simulink model "ClosedLoop"  (R2023b)
settings: Solver=ode1  StartTime=0.0  StopTime=inf  FixedStep=0.005  RelTol=1e-3  EnableMultiTasking=on
undefined symbols (not defined in the file or in its folder): Abar, Bbar, Cbar, F, G, Lbar
libraries: arduinolib x2, simulink x2
settings Model: SimulationMode=external  ExtModeTrigDuration=2  Creator=Alex  LastModifiedBy=jose
settings SolverCC: AlgebraicLoopSolver=TrustRegion
settings DataIOCC: SaveFormat=StructureWithTime  ReturnWorkspaceOutputs=off
settings OptimizationCC: PassReuseOutputArgsAs=Individual arguments  MaxStackSize=64  EfficientTunableParamExpr=on
settings DebuggingCC: ParameterTunabilityLossMsg=error  UnconnectedInputMsg=warning  UnconnectedOutputMsg=warning  UnconnectedLineMsg=warning  ArithmeticOperatorsInVariantConditions=warning
settings HardwareCC: ProdBitPerInt=16  ProdBitPerPointer=16  ProdBitPerSizeT=16  ProdBitPerPtrDiffT=16  ProdLargestAtomicFloat=None  ProdWordSize=8  ProdHWDeviceType=Atmel->AVR
settings ModelReferenceCC: EnableRefExpFcnMdlSchedulingChecks=on
settings SFSimCC: SimUseLocalCustomCode=off  MATLABDynamicMemAlloc=off  CustomCodeUndefinedFunction=UseInterfaceOnly
settings RTWCC: Description=Embedded Coder  SystemTargetFile=ert.tlc  HardwareBoard=Arduino Mega 2560  TemplateMakefile=ert_default_tmf  RTWUseLocalCustomCode=off  Toolchain=Arduino AVR  BuildConfiguration=Faster Runs  IncludeHyperlinkInReport=on  DLArmComputeVersion=19.05
settings CodeAppCC: ForceParamTrailComments=on  IgnoreCustomStorageClasses=off  OperatorAnnotations=on  SimulinkDataObjDesc=on  SFDataObjDesc=on  InsertBlockDesc=on
settings ERTTargetCC: SupportContinuousTime=on  SupportVariableSizeSignals=on  ExtModeTransport=3  ExtModeStaticAlloc=on  ExtModeStaticAllocSize=1000  ExtModeMexFile=ext_xcp  ExtModeIntrfLevel=Level2 - Open

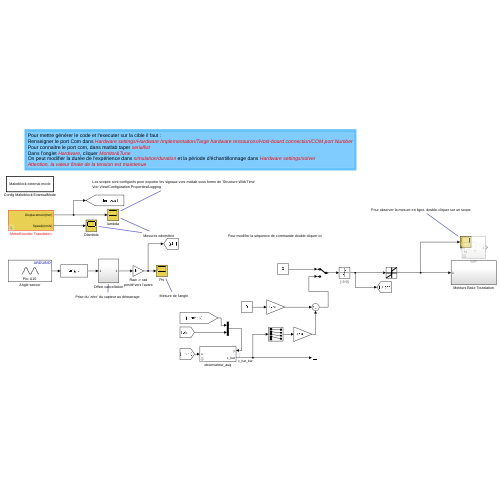
[thumbnail: Simulink's stored preview of the top-level diagram]
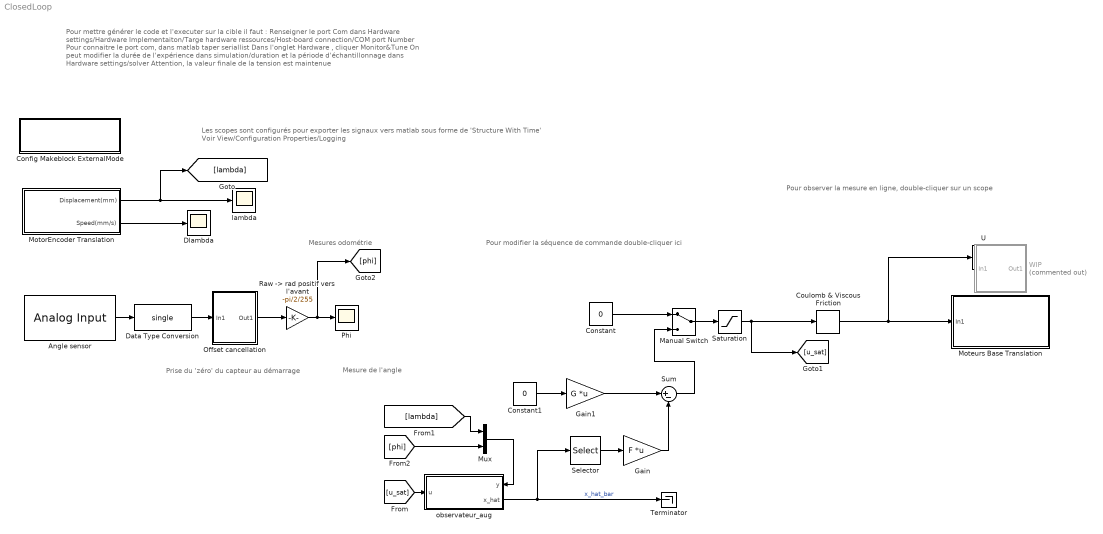
== system ClosedLoop ==
  note: Prise du 'zéro' du capteur au démarrage
  note: Mesure de l'angle
  note: Mesures odométrie
  note: Pour observer la mesure en ligne, double-cliquer sur un scope
  note: Pour modifier la séquence de commande double-cliquer ici
  note: Pour mettre générer le code et l'executer sur la cible il faut :
      | Renseigner le port Com dans Hardware settings/Hardware Implementaiton/Targe hardware ressources/Host-board connection/COM port Number
      | Pour connaitre le port com, dans matlab taper seriallist
      | Dans l'onglet Hardware , cliquer Monitor&Tune
      | On peut modifier la durée de l'expérience dans simulation/duration et la période d'échantillonnage dans Hardware settings/solver
      | Attention, la valeur finale de la tension est maintenue
  note: Les scopes sont configurés pour exporter les signaux vers matlab sous forme de 'Structure With Time'
      | Voir View/Configuration Properties/Logging
  Angle sensor : arduinolib/Analog Input  pinNumber=10  ReadResultsOnly=off  ConversionTriggerSource=Software  ExternalTriggerType=uint32(0)  OutputDataType=uint16  EnableConversionCompleteNotify=off  EnableOuputStatus=off  SampleTime=-1  blockPlatform=arduino
  Config Makeblock ExternalMode : Subsystem  LoadFcn=set_param(gcb,'MaskHideContents','on')  InitFcn=|  TreatAsAtomicUnit=on
      | codertarget.arduinobase.registry.setBaudRate(gcs,115200)
      | set_param(gcb,'MaskHideContents','on')
      mask Display: disp('Makeblock external mode')
  Constant : Constant  Value=0
  Constant1 : Constant  Value=0
  Coulomb & Viscous Friction : simulink/Discontinuities/Coulomb & Viscous Friction  offset=0.5  gain=1
  Data Type Conversion : DataTypeConversion  OutDataTypeStr=single  SaturateOnIntegerOverflow=off  RndMeth=Floor
  Dlambda : Scope
  Gain : Gain  Gain=F  Multiplication=Matrix(K*u)
  Gain1 : Gain  Gain=G  Multiplication=Matrix(K*u)
  Manual Switch : ManualSwitch
  Moteurs Base Translation : Subsystem
  MotorEncoder Translation : Subsystem  mask{pulsePerTurn=8, beltPitch=2.032, nTeeth=90, gearRatio=46}
      mask prompts: pulsePerTurn "Encoder resolution"; beltPitch "Belt Pitch"; nTeeth "Number of teeth"; gearRatio "Gear ratio"
  Mux : Mux  Inputs=2
  Offset cancellation : Subsystem
  Phi : Scope
  "Raw -> rad positif vers l'avant" : Gain  Gain=-pi/2/255
  Saturation : Saturate  UpperLimit=9  LowerLimit=-9
      settings: AttributesFormatString=[%<LowerLimit> %<UpperLimit>]
  Selector : Selector  InputPortWidth=5  IndexOptions=Index vector (dialog)  Indices=[1:4]  OutputSizes=1
  Sum : Sum  Inputs=|+-
  Terminator : Terminator
  U : Scope
  WIP : Subsystem  Commented=on
  lambda : Scope
  observateur_aug : Subsystem  mask{A=Abar, B=Bbar, C=Cbar, x_hat0=0, L=Lbar}
      mask prompts: A "Matrice A"; B "Matrice B"; C "Matrice C"; x_hat0 "Condition initiale"; L "gain L"
      settings: PortSchema="{\"entries\":[{\"content\":{\"sides\":[{\"content\":{\"connectorIds\":[\"In1\"]},\"type\":\"ConnectorPlacement.EquallySpacedRectSide\",\"uuid\":\"1c206b57-f343-4802-943f-f396b5f2fa44\"},{\"content\":{\"connectorIds\":[\"In2\",\"Out1\"],\"side\":\"RIGHT\"},\"type\":\"ConnectorPlacement.EquallySpacedRectSide\",\"uuid\":\"35da9abd-d6b1-4089-aae6-a46dbed03912\"},{\"content\":{\"connectorIds\":[],\"side\":\"TOP\"},\"type\":\"ConnectorPlacement.EquallySpacedRectSide\",\"uuid\":\"b9f72e83-9b94-44ec-a47d-5a0319960312\"}]},\"type\":\"ConnectorPlacement.EquallySpacedConnector\",\"uuid\":\"6461eadb-104c-4216-897a-8e335480794d\"}],\"packageUris\":[\"http://schema.mathworks.com/mf0/Connector/R2020b\"],\"version\":\"1.0\"}"
  wires:
  MotorEncoder Translation/1(Displacement(mm)) -> [lambda], lambda/1
  Saturation/1 -> [u_sat], Coulomb & Viscous Friction/1
  Constant/1 -> Manual Switch/1
  Angle sensor/1 -> Data Type Conversion/1
  Offset cancellation/1(Out1) -> "Raw -> rad positif vers l'avant"/1
  Data Type Conversion/1 -> Offset cancellation/1(In1)
  "Raw -> rad positif vers l'avant"/1 -> [phi], Phi/1
  MotorEncoder Translation/2(Speed(mm/s)) -> Dlambda/1
  Manual Switch/1 -> Saturation/1
  [u_sat] -> observateur_aug/1(u)
  [lambda] -> Mux/1
  [phi] -> Mux/2
  Mux/1 -> observateur_aug/2(y)
  observateur_aug/1(x_hat) -> Selector/1, Terminator/1  "x_hat_bar"
  Selector/1 -> Gain/1
  Gain1/1 -> Sum/1
  Constant1/1 -> Gain1/1
  Gain/1 -> Sum/2
  Sum/1 -> Manual Switch/2
  Coulomb & Viscous Friction/1 -> U/1, Moteurs Base Translation/1(In1)

== system ClosedLoop/Config Makeblock ExternalMode ==

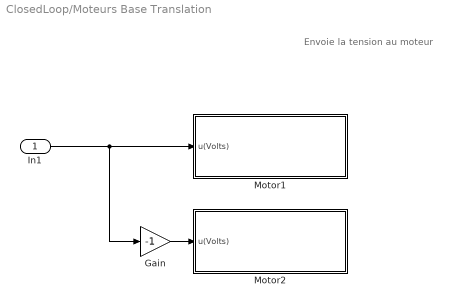
== system ClosedLoop/Moteurs Base Translation ==
  note: Envoie la tension au moteur
  In1 : Inport
  Gain : Gain  Gain=-1
  Motor1 : Subsystem  mask{Vmax=12}
      mask prompts: Vmax "Power supply Voltage"
  Motor2 : Subsystem  mask{Vmax=12}
      mask prompts: Vmax "Power supply Voltage"
  wires:
  Gain/1 -> Motor2/1(u(Volts))
  In1/1 -> Gain/1, Motor1/1(u(Volts))

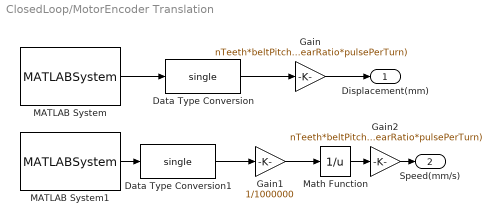
== system ClosedLoop/MotorEncoder Translation ==
  Data Type Conversion : DataTypeConversion  OutDataTypeStr=single  SaturateOnIntegerOverflow=off  RndMeth=Floor
  Data Type Conversion1 : DataTypeConversion  OutDataTypeStr=single  SaturateOnIntegerOverflow=off  RndMeth=Floor
  Gain : Gain  Gain=nTeeth*beltPitch/(gearRatio*pulsePerTurn)  OutDataTypeStr=single
      settings: AttributesFormatString=%<Gain>
  Gain1 : Gain  Gain=1/1000000
  Gain2 : Gain  Gain=nTeeth*beltPitch/(gearRatio*pulsePerTurn)  OutDataTypeStr=single
      settings: AttributesFormatString=%<Gain>
  MATLAB System : MATLABSystem  System=Enc1Read  SampleTime=-1
      mask Type: Enc1Read
      mask Display:
      | disp('Encoder 1');
      | port_label('output',1,'y');
  MATLAB System1 : MATLABSystem  System=Enc1Period  SampleTime=-1
      mask Type: Enc1Period
      mask Display:
      | disp('Encoder Period 1');
      | port_label('output',1,'y');
  Math Function : Math  Operator=reciprocal  SignedPower=on  OutputSignalType=real  OutDataTypeStr=single  SaturateOnIntegerOverflow=off
  Displacement(mm) : Outport  VectorParamsAs1DForOutWhenUnconnected=off
  Speed(mm/s) : Outport  Port=2  VectorParamsAs1DForOutWhenUnconnected=off
  wires:
  MATLAB System/1 -> Data Type Conversion/1
  Gain/1 -> Displacement(mm)/1
  Data Type Conversion/1 -> Gain/1
  Gain1/1 -> Math Function/1
  Data Type Conversion1/1 -> Gain1/1
  MATLAB System1/1 -> Data Type Conversion1/1
  Math Function/1 -> Gain2/1
  Gain2/1 -> Speed(mm/s)/1

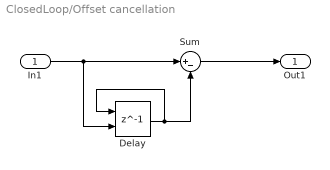
== system ClosedLoop/Offset cancellation ==
  In1 : Inport
  Delay : Delay  DelayLength=1  InitialConditionSource=Input port
      settings: InputPortMap=u0,p4
  Sum : Sum  Inputs=|+-
  Out1 : Outport  VectorParamsAs1DForOutWhenUnconnected=off
  wires:
  In1/1 -> Sum/1, Delay/2
  Delay/1 -> Sum/2, Delay/1
  Sum/1 -> Out1/1

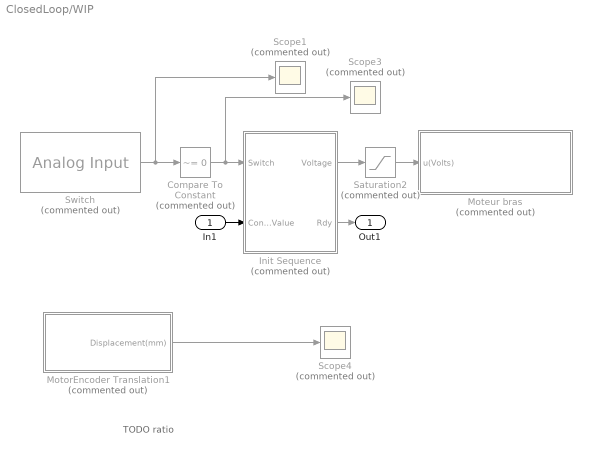
== system ClosedLoop/WIP ==
  note: TODO ratio
  In1 : Inport
  Compare To Constant : simulink/Logic and Bit Operations/Compare To Constant  Commented=on  relop=~=  const=0  OutDataTypeStr=boolean
  Init Sequence : Stateflow chart  Commented=on  TreatAsAtomicUnit=on
  Moteur bras : Subsystem  Commented=on  mask{Vmax=12}
      mask prompts: Vmax "Power supply Voltage"
  MotorEncoder Translation1 : Subsystem  Commented=on  mask{pulsePerTurn=8, beltPitch=2.032, nTeeth=90, gearRatio=46}
      mask prompts: pulsePerTurn "Encoder resolution"; beltPitch "Belt Pitch"; nTeeth "Number of teeth"; gearRatio "Gear ratio"
  Saturation2 : Saturate  Commented=on  UpperLimit=9  LowerLimit=-9
      settings: AttributesFormatString=[%<LowerLimit> %<UpperLimit>]
  Scope1 : Scope  Commented=on
  Scope3 : Scope  Commented=on
  Scope4 : Scope  Commented=on
  Switch : arduinolib/Analog Input  Commented=on  pinNumber=11  ReadResultsOnly=off  ConversionTriggerSource=Software  ExternalTriggerType=uint32(0)  OutputDataType=uint16  EnableConversionCompleteNotify=off  EnableOuputStatus=off  SampleTime=-1  blockPlatform=arduino
  Out1 : Outport
  wires:
  In1/1 -> Init Sequence/2(ControlValue)
  Init Sequence/1(Voltage) -> Saturation2/1
  Init Sequence/2(Rdy) -> Out1/1
  Switch/1 -> Scope1/1, Compare To Constant/1
  Compare To Constant/1 -> Scope3/1, Init Sequence/1(Switch)
  MotorEncoder Translation1/1(Displacement(mm)) -> Scope4/1
  Saturation2/1 -> Moteur bras/1(u(Volts))

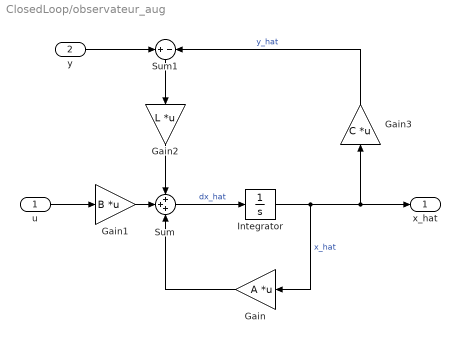
== system ClosedLoop/observateur_aug ==
  u : Inport
  y : Inport  Port=2
  Gain : Gain  Gain=A  Multiplication=Matrix(K*u)
  Gain1 : Gain  Gain=B  Multiplication=Matrix(K*u)
  Gain2 : Gain  Gain=L  Multiplication=Matrix(K*u)
  Gain3 : Gain  Gain=C  Multiplication=Matrix(K*u)
  "Integrator " : Integrator  InitialCondition=x_hat0
  Sum : Sum  Inputs=+++
  Sum1 : Sum  Inputs=+-
  x_hat : Outport
  wires:
  Gain3/1 -> Sum1/2  "y_hat"
  Sum1/1 -> Gain2/1
  y/1 -> Sum1/1
  Gain2/1 -> Sum/1
  u/1 -> Gain1/1
  Gain1/1 -> Sum/2
  Gain/1 -> Sum/3
  "Integrator "/1 -> Gain/1, x_hat/1, Gain3/1  "x_hat"
  Sum/1 -> "Integrator "/1  "dx_hat"

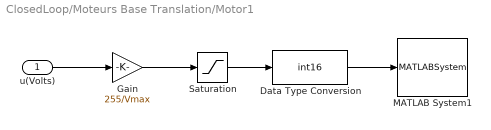
== system ClosedLoop/Moteurs Base Translation/Motor1 ==
  u(Volts) : Inport
  Data Type Conversion : DataTypeConversion  OutDataTypeStr=int16  SaturateOnIntegerOverflow=off  RndMeth=Floor
  Gain : Gain  Gain=255/Vmax
      settings: AttributesFormatString=%<Gain>
  MATLAB System1 : MATLABSystem  System=DCMotor1Set
      mask Type: DCMotor1Set
      mask Display:
      | disp('DC Motor 1');
      | port_label('input',1,'u');
  Saturation : Saturate  UpperLimit=255  LowerLimit=-255
  wires:
  Gain/1 -> Saturation/1
  u(Volts)/1 -> Gain/1
  Data Type Conversion/1 -> MATLAB System1/1
  Saturation/1 -> Data Type Conversion/1

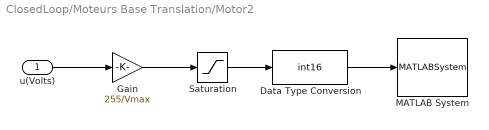
== system ClosedLoop/Moteurs Base Translation/Motor2 ==
  u(Volts) : Inport
  Data Type Conversion : DataTypeConversion  OutDataTypeStr=int16  SaturateOnIntegerOverflow=off  RndMeth=Floor
  Gain : Gain  Gain=255/Vmax
      settings: AttributesFormatString=%<Gain>
  MATLAB System : MATLABSystem  System=DCMotor2Set
      mask Type: DCMotor2Set
      mask Display:
      | disp('DC Motor 2');
      | port_label('input',1,'u');
  Saturation : Saturate  UpperLimit=255  LowerLimit=-255
  wires:
  Saturation/1 -> Data Type Conversion/1
  Data Type Conversion/1 -> MATLAB System/1
  u(Volts)/1 -> Gain/1
  Gain/1 -> Saturation/1

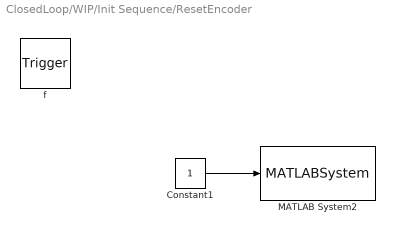
== system ClosedLoop/WIP/Init Sequence/ResetEncoder ==
  f : TriggerPort  TriggerType=function-call  VariantControl=(inherit)
      settings: CopyFcn=Stateflow.SLINSF.SimulinkMan.removeBlockPreDeleteFcn  PreDeleteFcn=Stateflow.SLINSF.SimulinkMan.unsafePredeleteFcn
  Constant1 : Constant  OutDataTypeStr=uint16
  MATLAB System2 : MATLABSystem  System=EncReset  Port=3
      mask Type: EncReset
      mask Display:
      | disp('Enc Reset 3');
      | port_label('input',1,'u');
  wires:
  Constant1/1 -> MATLAB System2/1

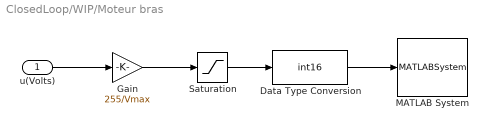
== system ClosedLoop/WIP/Moteur bras ==
  u(Volts) : Inport
  Data Type Conversion : DataTypeConversion  OutDataTypeStr=int16  SaturateOnIntegerOverflow=off  RndMeth=Floor
  Gain : Gain  Gain=255/Vmax
      settings: AttributesFormatString=%<Gain>
  MATLAB System : MATLABSystem  System=DCMotor3Set
      mask Type: DCMotor3Set
      mask Display:
      | disp('DC Motor 3');
      | port_label('input',1,'u');
  Saturation : Saturate  UpperLimit=255  LowerLimit=-255
  wires:
  Gain/1 -> Saturation/1
  u(Volts)/1 -> Gain/1
  Data Type Conversion/1 -> MATLAB System/1
  Saturation/1 -> Data Type Conversion/1

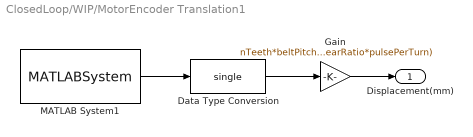
== system ClosedLoop/WIP/MotorEncoder Translation1 ==
  Data Type Conversion : DataTypeConversion  OutDataTypeStr=single  SaturateOnIntegerOverflow=off  RndMeth=Floor
  Gain : Gain  Gain=nTeeth*beltPitch/(gearRatio*pulsePerTurn)  OutDataTypeStr=single
      settings: AttributesFormatString=%<Gain>
  MATLAB System1 : MATLABSystem  System=Enc3Read  SampleTime=-1
      mask Type: Enc3Read
      mask Display:
      | disp('Encoder 3');
      | port_label('output',1,'y');
  Displacement(mm) : Outport  VectorParamsAs1DForOutWhenUnconnected=off
  wires:
  Data Type Conversion/1 -> Gain/1
  Gain/1 -> Displacement(mm)/1
  MATLAB System1/1 -> Data Type Conversion/1

== stateflow chart ClosedLoop/WIP/Init Sequence ==
  state ResetEncoder [function]
  state Homing
    during:
    Voltage = -1.4;
  state LeavingZero
    during:
    Voltage = 1.4;
  state Ready
    entry:
    Rdy = 1;
    during:
    Voltage = ControlValue;
    exit:
    Rdy=0;
  (default) -> Homing
  Homing -> LeavingZero : [Switch>0]
  Ready -> LeavingZero : [Switch>0]
  LeavingZero -> Ready : [Switch==0]{ResetEncoder()}
  data: Switch input; ControlValue input; Voltage output; Rdy output
